simulink model "zadanie4STPRYS"  (R2014b)
settings: Solver=ode45  StartTime=0.0  StopTime=60  RelTol=1e-3
values from neighbouring files (symbols this model uses):
  T = 0.5    [zadanie1STP.m]
settings Model: Creator=KonradSob  LastModifiedBy=KonradSob

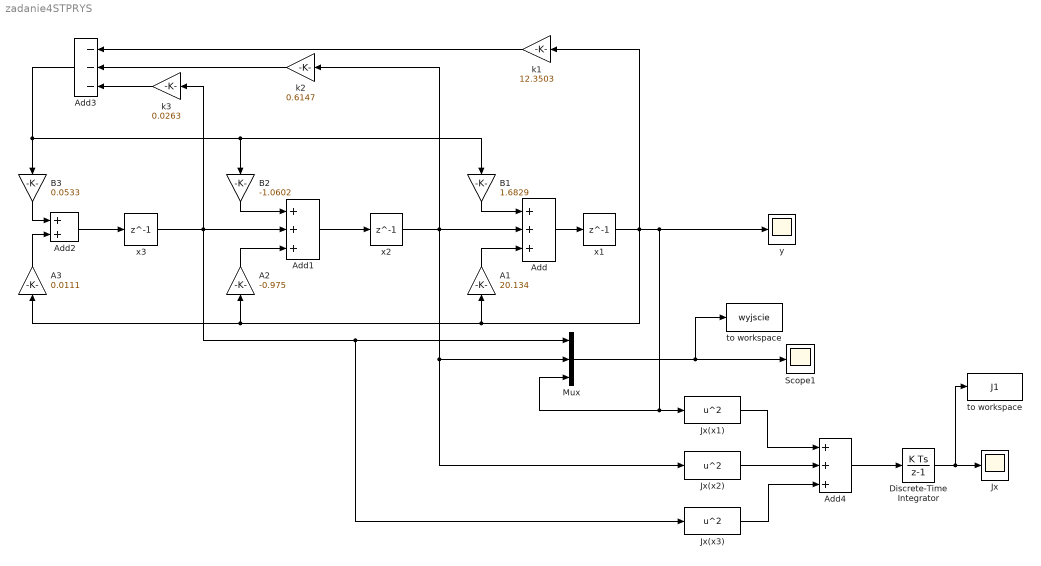
== system zadanie4STPRYS ==
  A1 : Gain  Gain=20.134
  A2 : Gain  Gain=-0.975
  A3 : Gain  Gain=0.0111
  Add : Sum  Inputs=+++
  Add1 : Sum  Inputs=+++
  Add2 : Sum
  Add3 : Sum  Inputs=---
  Add4 : Sum  Inputs=+++
  B1 : Gain  Gain=1.6829
  B2 : Gain  Gain=-1.0602
  B3 : Gain  Gain=0.0533
  Discrete-Time Integrator : DiscreteIntegrator  gainval=1/12  InitialConditionSetting=State (most efficient)
  Jx : Scope
      settings: SaveName=ScopeData2
  Jx(x1) : Fcn  Expr=u^2
  Jx(x2) : Fcn  Expr=u^2
  Jx(x3) : Fcn  Expr=u^2
  Mux : Mux  Inputs=3
  Scope1 : Scope
  k1 : Gain  Gain=12.3503
  k2 : Gain  Gain=0.6147
  k3 : Gain  Gain=0.0263
  to workspace : ToWorkspace  VariableName=J1  SaveFormat=Timeseries  SampleTime=-1
  "to workspace " : ToWorkspace  VariableName=wyjscie  SaveFormat=Timeseries  SampleTime=-1
  x1 : Delay  DelayLength=1  InitialCondition=5  SampleTime=T
  x2 : Delay  DelayLength=1  InitialCondition=-1  SampleTime=T
  x3 : Delay  DelayLength=1  InitialCondition=3  SampleTime=T
  y : Scope
      settings: YMin=4  YMax=6
  wires:
  x1/1 -> A3/1, A2/1, A1/1, Jx(x1)/1, Mux/3, y/1, k1/1
  x2/1 -> Jx(x2)/1, Mux/2, Add/2, k2/1
  Add/1 -> x1/1
  Add2/1 -> x3/1
  Add1/1 -> x2/1
  x3/1 -> Jx(x3)/1, Mux/1, Add1/2, k3/1
  k3/1 -> Add3/3
  k1/1 -> Add3/1
  Add3/1 -> B2/1, B1/1, B3/1
  B2/1 -> Add1/1
  Mux/1 -> "to workspace "/1, Scope1/1
  A3/1 -> Add2/2
  k2/1 -> Add3/2
  B1/1 -> Add/1
  A1/1 -> Add/3
  Jx(x1)/1 -> Add4/1
  Jx(x2)/1 -> Add4/2
  Jx(x3)/1 -> Add4/3
  Add4/1 -> Discrete-Time Integrator/1
  Discrete-Time Integrator/1 -> to workspace/1, Jx/1
  A2/1 -> Add1/3
  B3/1 -> Add2/1
